simulink model "CharacterizeMotorMC4_0"  (R2023a)
settings: Solver=FixedStepDiscrete  StartTime=0.0  StopTime=256  FixedStep=6.35  RelTol=1e-3  EnableMultiTasking=on
model workspace (MAT data in the model file):
  M5_motor = 0
  s = 0.01
libraries: arduinolib x8, simulink x2, eeGeneralControl x2, SignalEditorBlockLib x1
settings Model: ExtModeTrigDuration=2  Creator=auw_a  LastModifiedBy=auw_a
settings OptimizationCC: EnhancedBackFolding=on  PassReuseOutputArgsAs=Individual arguments  ZeroExternalMemoryAtStartup=off  ZeroInternalMemoryAtStartup=off  MaxStackSize=64  OptimizeBlockOrder=speed  DifferentSizesBufferReuse=on  OptimizationCustomize=off  EfficientTunableParamExpr=on
settings DebuggingCC: ParameterTunabilityLossMsg=error
settings HardwareCC: ProdBitPerPointer=32  ProdBitPerSizeT=32  ProdBitPerPtrDiffT=32  ProdLargestAtomicInteger=Long  ProdLargestAtomicFloat=Double  ProdWordSize=32  ProdHWDeviceType=ARM Compatible->ARM Cortex
settings SFSimCC: MATLABDynamicMemAlloc=off
settings RTWCC: Description=Embedded Coder  SystemTargetFile=ert.tlc  HardwareBoard=ESP32-WROOM(Arduino Compatible)  TLCOptions="-aInlineSetEventsForThisBaseRateFcn=TLC_FALSE -aSuppressMultiTaskScheduler=TLC_FALSE  -aRateBasedStepFcn=0"  TemplateMakefile=ert_default_tmf  Toolchain=ESP32  BuildConfiguration=Faster Runs
settings CodeAppCC: ForceParamTrailComments=on  IgnoreCustomStorageClasses=off  OperatorAnnotations=on  SimulinkDataObjDesc=on  SFDataObjDesc=on  InsertBlockDesc=on
settings ERTTargetCC: SupportContinuousTime=on  SupportVariableSizeSignals=on  ExtModeTransport=3  ExtModeStaticAlloc=on  ExtModeAutomaticAllocSize=off  ExtModeStaticAllocSize=65536  ExtModeMexFile=ext_xcp  ExtModeIntrfLevel=Level2 - Open

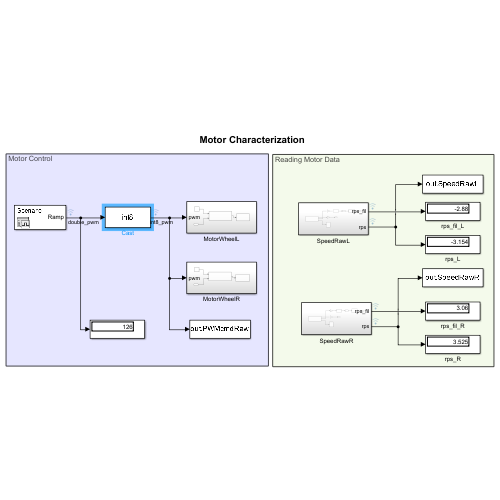
[thumbnail: Simulink's stored preview of the top-level diagram]
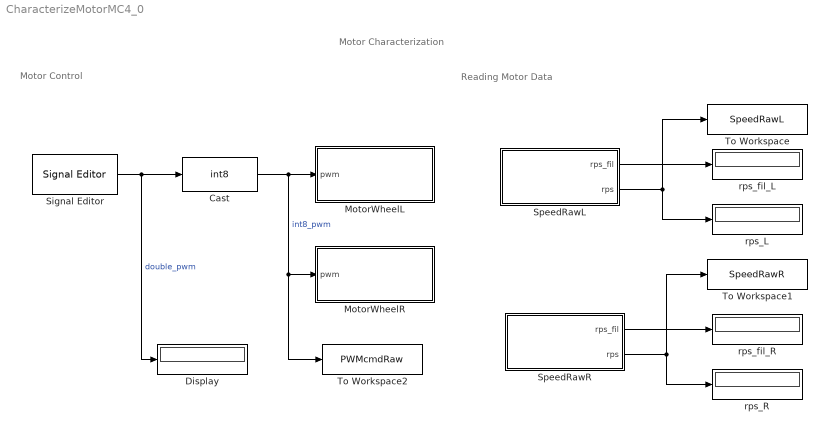
== system CharacterizeMotorMC4_0 ==
  note: Motor Characterization
  note: Motor Control
  note: Reading Motor Data
  Cast : DataTypeConversion  OutDataTypeStr=int8  SaturateOnIntegerOverflow=off  RndMeth=Floor
  Display : Display
  MotorWheelL : Subsystem
  MotorWheelR : Subsystem
  Signal Editor : SignalEditorBlockLib/Signal Editor  FileName=C:\Users\auw_a\Documents\MC4.0\MATLAB Workspace\CharacterizeMotorRampSignal.mat  ActiveScenario=Scenario  ActiveSignal=Ramp  IsBus=off  OutputBusObjectStr=Bus: BusObject  SampleTime=6.35  ZeroCross=off  OutputAfterFinalValue=Setting to zero  Unit=inherit  PreserveSignalName=on  ApplySigPropsToAllScenarios=on
  SpeedRawL : Subsystem
  SpeedRawR : Subsystem
  To Workspace : ToWorkspace  VariableName=SpeedRawL  SampleTime=-1
      settings: Save2DSignal=2-D array (concatenate along first dimension)
  To Workspace1 : ToWorkspace  VariableName=SpeedRawR  SampleTime=-1
      settings: Save2DSignal=2-D array (concatenate along first dimension)
  To Workspace2 : ToWorkspace  VariableName=PWMcmdRaw  SampleTime=-1
      settings: Save2DSignal=2-D array (concatenate along first dimension)
  rps_L : Display
  rps_R : Display
  rps_fil_L : Display
  rps_fil_R : Display
  wires:
  SpeedRawL/1(rps_fil) -> rps_fil_L/1
  SpeedRawL/2(rps) -> To Workspace/1, rps_L/1
  SpeedRawR/2(rps) -> To Workspace1/1, rps_R/1
  SpeedRawR/1(rps_fil) -> rps_fil_R/1
  Cast/1 -> To Workspace2/1, MotorWheelR/1(pwm), MotorWheelL/1(pwm)  "int8_pwm"
  Signal Editor/1 -> Display/1, Cast/1  "double_pwm"

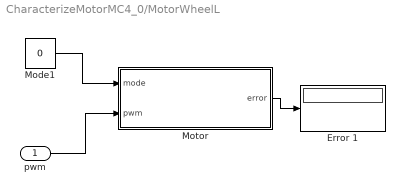
== system CharacterizeMotorMC4_0/MotorWheelL ==
  pwm : Inport
  Error 1 : Display
  Mode1 : Constant  Value=0
  Motor : Subsystem  mask(Encoder DC Motor){M5_motor=M1, error_select=on}
      mask prompts: M5_motor "Motor Port:"; error_select "Show error output port"
      mask help:
      | Set the speed and direction of the DC motor on the selected port.
      |
      | The block accepts an input between 127 to -127:
      | * 127 = Full speed forward
      | * 0 = Stop
      | * -127 = Full speed reverse
      mask init:
      | switch M5_motor
      |     case 'M1'
      |         m = 0;
      |     case 'M2'
      |         m = 1;
      |     case 'M3'
      |         m = 2;
      |     case 'M4'
      |         m = 3;
      | end
      | str = "Motor " + M5_motor;
      | label = str;
      mask Help:
      | The Motor DC Motors block controls the speed and direction of a DC motor connected to a MC4.0. The input signal determines the power supplied to the motor and the direction of rotation of the motor.
      | 
      | Supported Hardware
      | You can use the M1 M2 M3 M4 DC Motors block only with MC4.0 4Encoder Motor Module
      | 
      | PORTS
      | 
      | Input Port:
      | The sign of the input signal determines the direction of rotation of the DC motor. A positive sign indicates a forward rotation, whereas a negative sign indicates a reverse rotation. The amplitude determines the power supplied to the motor.
      | 
      | 1 to 127: Forward rotation, minimum to maximum power.
      | 
      | –1 to –127: Reverse rotation, minimum to maximum power.
      | 
      | 0: Stop.
      | 
      | Output Port:
      | [2x1] array
      | Indicates that the block outputs the status of the I2C write operation at the output port. One for mode and other for pwm.
      | The block outputs the status as a uint8 value. Each value corresponds to a data transfer status.
      | 
      | PARAMETERS
      | 
      | M5_motor - Port number on 4 Encoder Motor Module
      | M1 (default) | M2 | M3 | M4
      | Select the port number on the 4 Encoder Motor Module to which the DC motor is connected.
      mask TypeOptions M5_motor: M1 | M2 | M3 | M4
      mask Display:
      | im = imread('4EncoderMotorModule.jpg');
      | image(im, [40, 5, 50, 50]);
      | color('blue');
      | text(85, 10, label);
  wires:
  Motor/1(error) -> Error 1/1
  Mode1/1 -> Motor/1(mode)
  pwm/1 -> Motor/2(pwm)

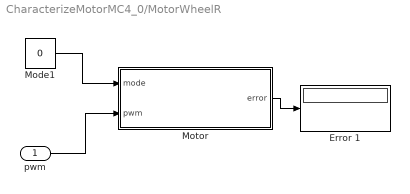
== system CharacterizeMotorMC4_0/MotorWheelR ==
  pwm : Inport
  Error 1 : Display
  Mode1 : Constant  Value=0
  Motor : Subsystem  mask(Encoder DC Motor){M5_motor=M2, error_select=on}
      mask prompts: M5_motor "Motor Port:"; error_select "Show error output port"
      mask help:
      | Set the speed and direction of the DC motor on the selected port.
      |
      | The block accepts an input between 127 to -127:
      | * 127 = Full speed forward
      | * 0 = Stop
      | * -127 = Full speed reverse
      mask init:
      | switch M5_motor
      |     case 'M1'
      |         m = 0;
      |     case 'M2'
      |         m = 1;
      |     case 'M3'
      |         m = 2;
      |     case 'M4'
      |         m = 3;
      | end
      | str = "Motor " + M5_motor;
      | label = str;
      mask Help:
      | The Motor DC Motors block controls the speed and direction of a DC motor connected to a MC4.0. The input signal determines the power supplied to the motor and the direction of rotation of the motor.
      | 
      | Supported Hardware
      | You can use the M1 M2 M3 M4 DC Motors block only with MC4.0 4Encoder Motor Module
      | 
      | PORTS
      | 
      | Input Port:
      | The sign of the input signal determines the direction of rotation of the DC motor. A positive sign indicates a forward rotation, whereas a negative sign indicates a reverse rotation. The amplitude determines the power supplied to the motor.
      | 
      | 1 to 127: Forward rotation, minimum to maximum power.
      | 
      | –1 to –127: Reverse rotation, minimum to maximum power.
      | 
      | 0: Stop.
      | 
      | Output Port:
      | [2x1] array
      | Indicates that the block outputs the status of the I2C write operation at the output port. One for mode and other for pwm.
      | The block outputs the status as a uint8 value. Each value corresponds to a data transfer status.
      | 
      | PARAMETERS
      | 
      | M5_motor - Port number on 4 Encoder Motor Module
      | M1 (default) | M2 | M3 | M4
      | Select the port number on the 4 Encoder Motor Module to which the DC motor is connected.
      mask TypeOptions M5_motor: M1 | M2 | M3 | M4
      mask Display:
      | im = imread('4EncoderMotorModule.jpg');
      | image(im, [40, 5, 50, 50]);
      | color('blue');
      | text(85, 10, label);
  wires:
  pwm/1 -> Motor/2(pwm)
  Mode1/1 -> Motor/1(mode)
  Motor/1(error) -> Error 1/1

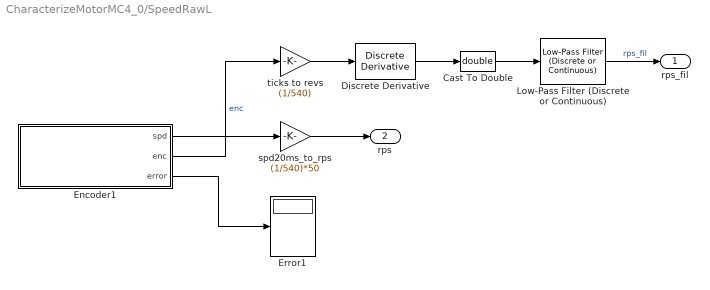
== system CharacterizeMotorMC4_0/SpeedRawL ==
  Cast To Double : DataTypeConversion  OutDataTypeStr=double  SaturateOnIntegerOverflow=off  RndMeth=Floor
  Discrete Derivative : simulink/Discrete/Discrete Derivative  gainval=1.0  ICPrevScaledInput=0.0  OutMin=[]  OutMax=[]  OutDataType=fixdt(1, 16)  OutScaling=2^-10  DoSatur=off
  Encoder1 : Subsystem  mask(Encoder - 4 Encoder DC Motor){M5_motor=1, s=6.35}
      mask prompts: M5_motor "Encoder channel:"; s "Sample Time:"
      mask help:
      | Measure the rotation of a motor in ticks.
      |
      | The block outputs the position and rotational speed of the motor. The position is measured in ticks and the speed is measured in ticks per 20ms of int32 data type.
      |
      | Every increment in the tick count indicates a clockwise rotation and every decrement in the tick count indicates a counterclockwise rotation.
      mask init:
      | switch M5_motor
      |     case '1'
      |         m = 0;
      |     case '2'
      |         m = 1;
      |     case '3'
      |         m = 2;
      |     case '4'
      |         m = 3;
      | end
      | str = "Encoder " + M5_motor;
      | label = str;
      mask Help:
      | PORTS
      | 
      | Output
      | 
      | Position - Position of rotating motor
      | scalar
      | The Position port outputs the relative change in the position of the rotating motor, measured in ticks.
      | Data Types: int32
      | 
      | Speed - Speed of rotating motor
      | scalar
      | The Speed port outputs the rotational speed of the motor, measured in ticks per 20 milli second.
      | Dependencies:
      | The Speed port is available only when you select the Show Speed output port parameter.
      | Data Types: int32
      | 
      | Output Port:
      | [2x1] array
      | Indicates that the block outputs the status of the I2C read operation at the output port. One for speed per 20ms and other for number of ticks.
      | The block outputs the status as a uint8 value. Each value corresponds to a data transfer status.
      | 
      | PARAMETERS
      | 
      | Encoder - Encoder channel number
      | 1 (default) | 2 | 3 | 4
      | Select the channel number of the encoder that is connected to the 4Encoder Motor Module.
      | 
      | Sample Time  - Time interval to read value fro encoder
      | 0.01 (default) |  -1 | non-negative real value
      | Specify how often the block reads the tick count from the encoder, in seconds. When you specify this parameter as -1, Simulink determines the best sample time for the block based on the block context within the model.
      mask TypeOptions M5_motor: 1 | 2 | 3 | 4
      mask Display:
      | im = imread('4EncoderModule.jpg');
      | image(im, [20, 5, 50, 50]);
      | color('blue');
      | text(75, 10, label);
  Error1 : Display
  Low-Pass Filter (Discrete or Continuous) : eeGeneralControl/Low-Pass Filter (Discrete or Continuous)  K=1  T=0.25  B=inf  A=-inf  init_option=Inherited from block input  x0=0  Ts=-1
  spd20ms_to_rps : Gain  Gain=(1/540)*50
  ticks to revs : Gain  Gain=(1/540)
  rps_fil : Outport
  rps : Outport  Port=2
  wires:
  Encoder1/3(error) -> Error1/1
  Discrete Derivative/1 -> Cast To Double/1
  Cast To Double/1 -> Low-Pass Filter (Discrete or Continuous)/1
  Encoder1/2(enc) -> ticks to revs/1  "enc"
  Encoder1/1(spd) -> spd20ms_to_rps/1
  ticks to revs/1 -> Discrete Derivative/1
  Low-Pass Filter (Discrete or Continuous)/1 -> rps_fil/1  "rps_fil"
  spd20ms_to_rps/1 -> rps/1

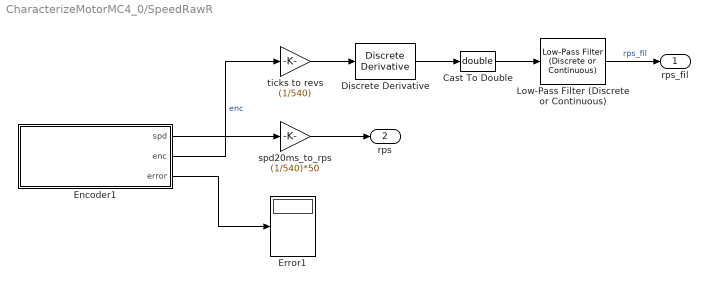
== system CharacterizeMotorMC4_0/SpeedRawR ==
  Cast To Double : DataTypeConversion  OutDataTypeStr=double  SaturateOnIntegerOverflow=off  RndMeth=Floor
  Discrete Derivative : simulink/Discrete/Discrete Derivative  gainval=1.0  ICPrevScaledInput=0.0  OutMin=[]  OutMax=[]  OutDataType=fixdt(1, 16)  OutScaling=2^-10  DoSatur=off
  Encoder1 : Subsystem  mask(Encoder - 4 Encoder DC Motor){M5_motor=2, s=6.35}
      mask prompts: M5_motor "Encoder channel:"; s "Sample Time:"
      mask help:
      | Measure the rotation of a motor in ticks.
      |
      | The block outputs the position and rotational speed of the motor. The position is measured in ticks and the speed is measured in ticks per 20ms of int32 data type.
      |
      | Every increment in the tick count indicates a clockwise rotation and every decrement in the tick count indicates a counterclockwise rotation.
      mask init:
      | switch M5_motor
      |     case '1'
      |         m = 0;
      |     case '2'
      |         m = 1;
      |     case '3'
      |         m = 2;
      |     case '4'
      |         m = 3;
      | end
      | str = "Encoder " + M5_motor;
      | label = str;
      mask Help:
      | PORTS
      | 
      | Output
      | 
      | Position - Position of rotating motor
      | scalar
      | The Position port outputs the relative change in the position of the rotating motor, measured in ticks.
      | Data Types: int32
      | 
      | Speed - Speed of rotating motor
      | scalar
      | The Speed port outputs the rotational speed of the motor, measured in ticks per 20 milli second.
      | Dependencies:
      | The Speed port is available only when you select the Show Speed output port parameter.
      | Data Types: int32
      | 
      | Output Port:
      | [2x1] array
      | Indicates that the block outputs the status of the I2C read operation at the output port. One for speed per 20ms and other for number of ticks.
      | The block outputs the status as a uint8 value. Each value corresponds to a data transfer status.
      | 
      | PARAMETERS
      | 
      | Encoder - Encoder channel number
      | 1 (default) | 2 | 3 | 4
      | Select the channel number of the encoder that is connected to the 4Encoder Motor Module.
      | 
      | Sample Time  - Time interval to read value fro encoder
      | 0.01 (default) |  -1 | non-negative real value
      | Specify how often the block reads the tick count from the encoder, in seconds. When you specify this parameter as -1, Simulink determines the best sample time for the block based on the block context within the model.
      mask TypeOptions M5_motor: 1 | 2 | 3 | 4
      mask Display:
      | im = imread('4EncoderModule.jpg');
      | image(im, [20, 5, 50, 50]);
      | color('blue');
      | text(75, 10, label);
  Error1 : Display
  Low-Pass Filter (Discrete or Continuous) : eeGeneralControl/Low-Pass Filter (Discrete or Continuous)  K=1  T=0.25  B=inf  A=-inf  init_option=Inherited from block input  x0=0  Ts=-1
  spd20ms_to_rps : Gain  Gain=(1/540)*50
  ticks to revs : Gain  Gain=(1/540)
  rps_fil : Outport
  rps : Outport  Port=2
  wires:
  spd20ms_to_rps/1 -> rps/1
  Low-Pass Filter (Discrete or Continuous)/1 -> rps_fil/1  "rps_fil"
  ticks to revs/1 -> Discrete Derivative/1
  Encoder1/1(spd) -> spd20ms_to_rps/1
  Encoder1/2(enc) -> ticks to revs/1  "enc"
  Cast To Double/1 -> Low-Pass Filter (Discrete or Continuous)/1
  Discrete Derivative/1 -> Cast To Double/1
  Encoder1/3(error) -> Error1/1

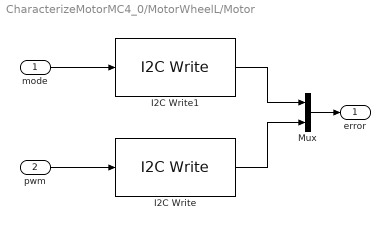
== system CharacterizeMotorMC4_0/MotorWheelL/Motor ==
  mode : Inport
  pwm : Inport  Port=2
  I2C Write : arduinolib/I2C Write  I2CModule=0  Mode=Master  SlaveAddress=uint8(hex2dec('24'))  SlaveByteOrder=BigEndian  Direction=Transmitter  RegisterAddressMode=on  RegisterAddress=uint8(hex2dec('20')) + m  SlaveDataType=uint8  DataLength=1  NoAck=off  RepeatedStart=off  OutputStatus=on  blockPlatform=ARDUINO
  I2C Write1 : arduinolib/I2C Write  I2CModule=0  Mode=Master  SlaveAddress=uint8(hex2dec('24'))  SlaveByteOrder=BigEndian  Direction=Transmitter  RegisterAddressMode=on  RegisterAddress=uint8(hex2dec('60')) + m  SlaveDataType=uint8  DataLength=1  NoAck=off  RepeatedStart=off  OutputStatus=on  blockPlatform=ARDUINO
  Mux : Mux  Inputs=2
  error : Outport
  wires:
  Mux/1 -> error/1
  I2C Write/1 -> Mux/2
  I2C Write1/1 -> Mux/1
  pwm/1 -> I2C Write/1
  mode/1 -> I2C Write1/1

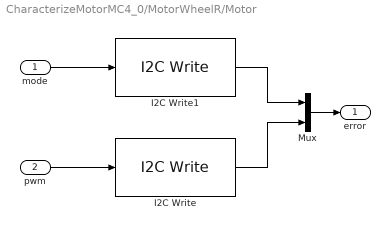
== system CharacterizeMotorMC4_0/MotorWheelR/Motor ==
  mode : Inport
  pwm : Inport  Port=2
  I2C Write : arduinolib/I2C Write  I2CModule=0  Mode=Master  SlaveAddress=uint8(hex2dec('24'))  SlaveByteOrder=BigEndian  Direction=Transmitter  RegisterAddressMode=on  RegisterAddress=uint8(hex2dec('20')) + m  SlaveDataType=uint8  DataLength=1  NoAck=off  RepeatedStart=off  OutputStatus=on  blockPlatform=ARDUINO
  I2C Write1 : arduinolib/I2C Write  I2CModule=0  Mode=Master  SlaveAddress=uint8(hex2dec('24'))  SlaveByteOrder=BigEndian  Direction=Transmitter  RegisterAddressMode=on  RegisterAddress=uint8(hex2dec('60')) + m  SlaveDataType=uint8  DataLength=1  NoAck=off  RepeatedStart=off  OutputStatus=on  blockPlatform=ARDUINO
  Mux : Mux  Inputs=2
  error : Outport
  wires:
  mode/1 -> I2C Write1/1
  pwm/1 -> I2C Write/1
  I2C Write1/1 -> Mux/1
  I2C Write/1 -> Mux/2
  Mux/1 -> error/1

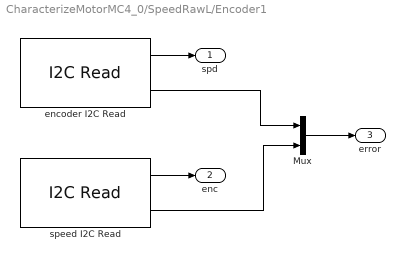
== system CharacterizeMotorMC4_0/SpeedRawL/Encoder1 ==
  Mux : Mux  Inputs=2
  encoder I2C Read : arduinolib/I2C Read  I2CModule=0  Mode=Master  SlaveAddress=uint8(hex2dec('24'))  SlaveByteOrder=BigEndian  Direction=Receiver  RegisterAddressMode=on  RegisterAddress=uint8(hex2dec('40')) + m  SlaveDataType=int8  DataLength=1  NoAck=off  RepeatedStart=off  OutputStatus=on  blockPlatform=ARDUINO  SampleTime=s
  speed I2C Read : arduinolib/I2C Read  I2CModule=0  Mode=Master  SlaveAddress=uint8(hex2dec('24'))  SlaveByteOrder=BigEndian  Direction=Receiver  RegisterAddressMode=on  RegisterAddress=uint8(hex2dec('30')) + 4*m  SlaveDataType=int32  DataLength=1  NoAck=off  RepeatedStart=off  OutputStatus=on  blockPlatform=ARDUINO  SampleTime=s
  spd : Outport
  enc : Outport  Port=2
  error : Outport  Port=3
  wires:
  Mux/1 -> error/1
  speed I2C Read/2 -> Mux/2
  encoder I2C Read/2 -> Mux/1
  speed I2C Read/1 -> enc/1
  encoder I2C Read/1 -> spd/1

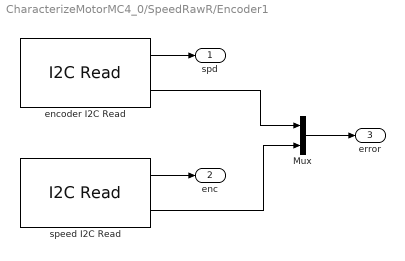
== system CharacterizeMotorMC4_0/SpeedRawR/Encoder1 ==
  Mux : Mux  Inputs=2
  encoder I2C Read : arduinolib/I2C Read  I2CModule=0  Mode=Master  SlaveAddress=uint8(hex2dec('24'))  SlaveByteOrder=BigEndian  Direction=Receiver  RegisterAddressMode=on  RegisterAddress=uint8(hex2dec('40')) + m  SlaveDataType=int8  DataLength=1  NoAck=off  RepeatedStart=off  OutputStatus=on  blockPlatform=ARDUINO  SampleTime=s
  speed I2C Read : arduinolib/I2C Read  I2CModule=0  Mode=Master  SlaveAddress=uint8(hex2dec('24'))  SlaveByteOrder=BigEndian  Direction=Receiver  RegisterAddressMode=on  RegisterAddress=uint8(hex2dec('30')) + 4*m  SlaveDataType=int32  DataLength=1  NoAck=off  RepeatedStart=off  OutputStatus=on  blockPlatform=ARDUINO  SampleTime=s
  spd : Outport
  enc : Outport  Port=2
  error : Outport  Port=3
  wires:
  encoder I2C Read/1 -> spd/1
  speed I2C Read/1 -> enc/1
  encoder I2C Read/2 -> Mux/1
  speed I2C Read/2 -> Mux/2
  Mux/1 -> error/1
